simulink model "SemCtrl_Art2012"  (R2021a)
settings: Solver=VariableStepAuto  StartTime=0.0  StopTime=30  RelTol=1e-3
settings Model: Creator=anira  LastModifiedBy=anira

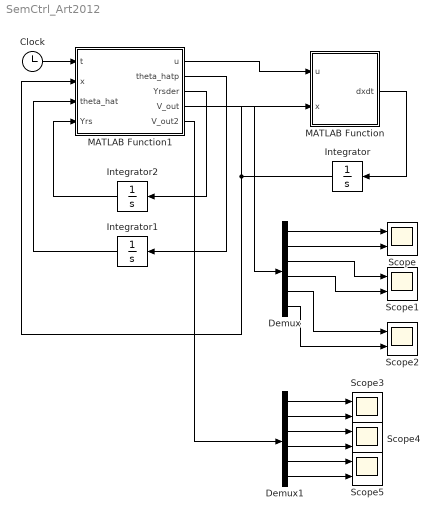
== system SemCtrl_Art2012 ==
  Clock : Clock
  Demux : Demux  Outputs=6
  Demux1 : Demux  Outputs=6
  Integrator : Integrator  InitialCondition=[0.5,-0.3,0.4]'
  Integrator1 : Integrator  InitialCondition=zeros(27,1)
  Integrator2 : Integrator  InitialCondition=[0.5,-0.3,0.4]'
  MATLAB Function : MATLAB Function  TreatAsAtomicUnit=on
  MATLAB Function1 : MATLAB Function  TreatAsAtomicUnit=on
  Scope{,1..5} (6 alike) : Scope  NumInputPorts=2
  wires:
  MATLAB Function/1(dxdt) -> Integrator/1
  Integrator/1 -> MATLAB Function1/2(x), MATLAB Function/2(x)
  MATLAB Function1/1(u) -> MATLAB Function/1(u)
  MATLAB Function1/2(theta_hatp) -> Integrator1/1
  Integrator1/1 -> MATLAB Function1/3(theta_hat)
  MATLAB Function1/3(Yrsder) -> Integrator2/1
  Integrator2/1 -> MATLAB Function1/4(Yrs)
  Clock/1 -> MATLAB Function1/1(t)
  MATLAB Function1/4(V_out) -> Demux/1
  Demux/1 -> Scope/1
  Demux/2 -> Scope/2
  Demux/3 -> Scope1/1
  Demux/4 -> Scope1/2
  Demux/5 -> Scope2/1
  Demux/6 -> Scope2/2
  MATLAB Function1/5(V_out2) -> Demux1/1
  Demux1/1 -> Scope3/1
  Demux1/2 -> Scope3/2
  Demux1/3 -> Scope4/1
  Demux1/4 -> Scope4/2
  Demux1/5 -> Scope5/1
  Demux1/6 -> Scope5/2

== matlab function SemCtrl_Art2012/MATLAB Function1 ==
  data: t input; u output; x input; theta_hatp output; theta_hat input; Yrs input; Yrsder output; V_out output; V_out2 output
function [u,theta_hatp,Yrsder,V_out,V_out2]= fcn(t,x,theta_hat,Yrs)

x1=x(1,1);
x2=x(2,1); 
x3=x(3,1);

Yr=Yrs(1,1);
Yrp=Yrs(2,1); 
Yr2p=Yrs(3,1);

yr=0.5*sin(t);
yrp=0.5*cos(t);
yr2p=-0.5*sin(t);
yr3p=-0.5*cos(t);
% --. Parametros del filtro.--
psi1=1; psi2=1; psi3=1;
omega1=1; omega2=1; omega3=1;
tau1=0.01; tau2=0.01; tau3=0.01;
T1=psi1*exp(-omega1*t)+tau1;
T2=psi2*exp(-omega2*t)+tau2;
T3=psi3*exp(-omega3*t)+tau3;
%T4=psi4*exp(-omega4*t)+tau4;

Yrsder=zeros(3,1);
Yrsder(1,1)=(yr-Yr)/T1;
Yrsder(2,1)=(yrp-Yrp)/T2;
Yrsder(3,1)=(yr2p-Yr2p)/T3;
%Yrsder(4,1)=(yr3p-Yr3p)/T4;
% --. Parametros de la RN
z1=x1-Yr;%1x1
xtilde=x1-Yr;
f1=x1^3;
x1p=x2+f1;
xtildep=x1p-yrp;

xx=[x1,x2,x3]';%Vector de entrada 3x1
c=[-0.5 -0.5 -0.5 -0.5 -0.5 -0.5 -0.5 -0.5 -0.5   0    0    0    0    0    0    0    0    0   0.5  0.5  0.5  0.5  0.5  0.5  0.5  0.5  0.5;        
   -0.5 -0.5 -0.5   0    0    0   0.5  0.5  0.5 -0.5 -0.5 -0.5   0    0    0   0.5  0.5  0.5 -0.5 -0.5 -0.5   0    0    0   0.5  0.5  0.5;
   -0.5   0   0.5 -0.5   0   0.5 -0.5   0   0.5 -0.5   0   0.5 -0.5   0   0.5 -0.5   0   0.5 -0.5   0   0.5 -0.5   0   0.5 -0.5   0   0.5];

mu=10; % Amplitud
sigma=20; % Ancho de funciones de activación

N=27;% No. de nodos
[aa,m]=size(c);% m=27
xi=zeros(m,1);
    for j=1:m
        c_j=c(:,j);% 2x1
        sigma_j=sigma;% 1x1
        xi(j,1)=mu*exp(-(norm(xx-c_j)^2/(sigma_j^2)));% Función de activación  mx1
    end

eta=0.5;Gamma=diag(4);
theta_hatp=Gamma*(z1*xi-eta*theta_hat);%3x1
F3_ast_est=theta_hat'*xi;
% --. Parámetros de control .--
k1=12; k2=10; k3=12;
K_31=k1+k2+k3;
K_32=k1*k2+k1*k3+k2*k3;
K_33=k1*k2*k3;
K_21=k1+k2;
K_22=k2*k1;

% % --. Ejemplo 1 .--
% f1=x1^3;
% f2=x1^2+x2^2;
% f3=0;
% parF1x1_as=3*x1^2;
% parF2x1_as=K_21*3*x1^2+2*x1+6*x2*x1+15*x1^4;
% parF2x2_as=2*x2+3*x1^2;
% F3=f3+K_21*f2+K_22*f1+parF2x1_as*(x2+f1)+parF2x2_as*(x3+f2);
% F2=f2+k1*f1+parF1x1_as*(x2+f1);
% F1_ast=f1;
% F2_ast=k2*F1_ast+F2;
% F3_ast=k3*F2_ast+F3; 

% --. Ejemplo 2 .--
f1=2*x1^2*sin(x2);
f2=x1^2+x1*x2+x2*cos(x1);
f3=x1*x3+x2^2+x3*sin(x2);
parF1x1_as=4*x1*sin(x2);
parF2x1_as=K_21*4*x1*sin(x2)+2*x1+x2-x2*sin(x1)+4*sin(x2)*(x2+2*x1^2*sin(x2))+4*x1*sin(x2)*(4*x1*sin(x2));
parF2x2_as=K_21*2*x1^2*cos(x2)+x1+cos(x1)+4*x1*cos(x2)*(x2+2*x1^2*sin(x2))+4*x1*sin(x2)*(1+2*x1^2*cos(x2));
F3=f3+K_21*f2+K_22*f1+parF2x1_as*(x2+f1)+parF2x2_as*(x3+f2);
F2=f2+k1*f1+parF1x1_as*(x2+f1);
F1_ast=f1;
F2_ast=k2*F1_ast+F2;
F3_ast=k3*F2_ast+F3; 

u=yr3p-K_31*(x3-Yr2p)-K_32*(x2-Yrp)-K_33*(x1-Yr)-theta_hat'*xi;%1x1
%u=Yr3p-K_31*(x3-Yr2p)-K_32*(x2-Yrp)-K_33*(x1-Yr)-F3_ast;%1x1

V_out=[ yr, x1,z1,u,F3_ast,F3_ast_est]';%5x1
V_out2=[ yr, Yr, yrp,Yrp,yr2p,Yr2p]';

== matlab function SemCtrl_Art2012/MATLAB Function ==
  data: u input; x input; dxdt output
function dxdt = fcn(u,x)
x1=x(1,1);
x2=x(2,1); 
x3=x(3,1);
% % --. Ejemplo1 .--
% f1=x1^3;
% f2=x1^2+x2^2;
% f3=0;
% --. Ejemplo2 .--
f1=2*x1^2*sin(x2);
f2=x1^2+x1*x2+x2*cos(x1);
f3=x1*x3+x2^2+x3*sin(x2);

dxdt=zeros(3,1);
dxdt(1,1)=x2+f1;
dxdt(2,1)=x3+f2;
dxdt(3,1)=u+f3;

% dxdt=zeros(3,1);
% dxdt(1,1)=x2;
% dxdt(2,1)=x3;
% dxdt(3,1)=u;
y=x1;
